simulink model "ltspidservo"  (Simulink 7.9)
settings: Solver=ode1  StartTime=0.0  StopTime=stoptime  FixedStep=(1/10000)  RelTol=1e-3
values from neighbouring files (symbols this model uses):
  Ap = [0              Cy           0          0 ... (first row only)    [LoadnCheckModel.m]
  Ayaw = [0            Cx        0           0 ... (first row only)    [LoadnCheckModel.m]
  Bp = [0 0 0 KsEL*CwEL/tausEL]'    [LoadnCheckModel.m]
  Byaw = [0     0    0   KsAZ*CwAZ/tausAZ]'    [LoadnCheckModel.m]
  Cp = [1 0 0 0]    [LoadnCheckModel.m]
  Cyaw = [1 0 0 0]    [LoadnCheckModel.m]
  dt = 0.0001    [main (ADMIN-PC's conflicted copy 2013-10-01).m]    (also in main.m)
  Gp = [0      1/Jey    0           0]'    [LoadnCheckModel.m]
  Gyaw = [0      1/Ja    0           0]'    [LoadnCheckModel.m]
  ref = 15.15    [main (ADMIN-PC's conflicted copy 2013-10-01).m]    (also in main.m)
  W = 1e-3    (= 0.001)    [main (ADMIN-PC's conflicted copy 2013-10-01).m]    (also in main.m; run_kCC.m = 1)
libraries: simulink x2
settings Model: Creator=Firdous  LastModifiedBy=ADMIN
settings DataIOCC: LimitDataPoints=off
settings GRTTargetCC: CombineOutputUpdateFcns=off  GRTInterface=on

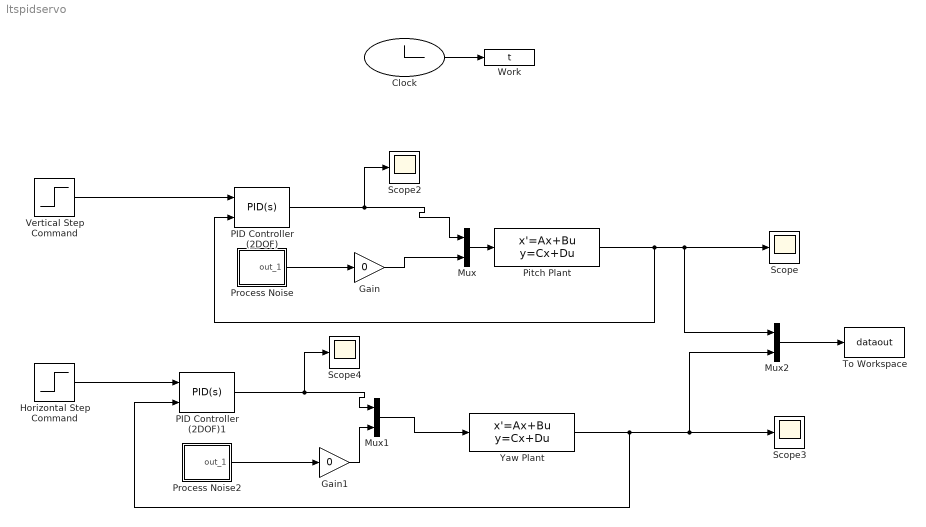
== system ltspidservo ==
  Clock : Clock
  Gain : Gain  Gain=0
  Gain1 : Gain  Gain=0
  Horizontal Step Command : Step  Time=0  After=15.15  SampleTime=0
  Mux : Mux  Inputs=2
  Mux1 : Mux  Inputs=2
  Mux2 : Mux  Inputs=2
  PID Controller (2DOF) : simulink/Continuous/PID Controller (2DOF)  Controller=PID  TimeDomain=Continuous-time  SampleTime=1  IntegratorMethod=Forward Euler  FilterMethod=Forward Euler  Form=Parallel  P=0.0314639161164997  I=0.00100652390344052  D=0.118069343591076  N=9.02659370005772  b=1  c=1  InitialConditionSource=internal  InitialConditionForIntegrator=0  InitialConditionForFilter=0  ExternalReset=none  LimitOutput=off  UpperSaturationLimit=inf  LowerSaturationLimit=-inf  LinearizeAsGain=off  AntiWindupMode=none  Kb=1  TrackingMode=off  Kt=1  PParamMin=[]  PParamMax=[]  IParamMin=[]  IParamMax=[]  DParamMin=[]  DParamMax=[]  NParamMin=[]  NParamMax=[]  bParamMin=[]  bParamMax=[]  cParamMin=[]  cParamMax=[]  KbParamMin=[]  KbParamMax=[]  KtParamMin=[]  KtParamMax=[]  POutMin=[]  POutMax=[]  IOutMin=[]  IOutMax=[]  DOutMin=[]  DOutMax=[]  NOutMin=[]  NOutMax=[]  bOutMin=[]  bOutMax=[]  cOutMin=[]  cOutMax=[]  KbOutMin=[]  KbOutMax=[]  KtOutMin=[]  KtOutMax=[]  IntegratorOutMin=[]  IntegratorOutMax=[]  FilterOutMin=[]  FilterOutMax=[]  SumOutMin=[]  SumOutMax=[]  Sum1OutMin=[]  Sum1OutMax=[]  Sum2OutMin=[]  Sum2OutMax=[]  Sum3OutMin=[]  Sum3OutMax=[]  SumI1OutMin=[]  SumI1OutMax=[]  SumI2OutMin=[]  SumI2OutMax=[]  SumI3OutMin=[]  SumI3OutMax=[]  SumDOutMin=[]  SumDOutMax=[]  SaturationOutMin=[]  SaturationOutMax=[]  IntegratorContinuousStateAttributes=''  IntegratorStateMustResolveToSignalObject=off  IntegratorRTWStateStorageClass=Auto  FilterContinuousStateAttributes=''  FilterStateMustResolveToSignalObject=off  FilterRTWStateStorageClass=Auto
  PID Controller (2DOF)1 : simulink/Continuous/PID Controller (2DOF)  Controller=PID  TimeDomain=Continuous-time  SampleTime=1  IntegratorMethod=Forward Euler  FilterMethod=Forward Euler  Form=Parallel  P=0.0104040475760461  I=0.000243006668049098  D=0.0472971950488125  N=6.44927650740255  b=1  c=1  InitialConditionSource=internal  InitialConditionForIntegrator=0  InitialConditionForFilter=0  ExternalReset=none  LimitOutput=off  UpperSaturationLimit=inf  LowerSaturationLimit=-inf  LinearizeAsGain=off  AntiWindupMode=none  Kb=1  TrackingMode=off  Kt=1  PParamMin=[]  PParamMax=[]  IParamMin=[]  IParamMax=[]  DParamMin=[]  DParamMax=[]  NParamMin=[]  NParamMax=[]  bParamMin=[]  bParamMax=[]  cParamMin=[]  cParamMax=[]  KbParamMin=[]  KbParamMax=[]  KtParamMin=[]  KtParamMax=[]  POutMin=[]  POutMax=[]  IOutMin=[]  IOutMax=[]  DOutMin=[]  DOutMax=[]  NOutMin=[]  NOutMax=[]  bOutMin=[]  bOutMax=[]  cOutMin=[]  cOutMax=[]  KbOutMin=[]  KbOutMax=[]  KtOutMin=[]  KtOutMax=[]  IntegratorOutMin=[]  IntegratorOutMax=[]  FilterOutMin=[]  FilterOutMax=[]  SumOutMin=[]  SumOutMax=[]  Sum1OutMin=[]  Sum1OutMax=[]  Sum2OutMin=[]  Sum2OutMax=[]  Sum3OutMin=[]  Sum3OutMax=[]  SumI1OutMin=[]  SumI1OutMax=[]  SumI2OutMin=[]  SumI2OutMax=[]  SumI3OutMin=[]  SumI3OutMax=[]  SumDOutMin=[]  SumDOutMax=[]  SaturationOutMin=[]  SaturationOutMax=[]  IntegratorContinuousStateAttributes=''  IntegratorStateMustResolveToSignalObject=off  IntegratorRTWStateStorageClass=Auto  FilterContinuousStateAttributes=''  FilterStateMustResolveToSignalObject=off  FilterRTWStateStorageClass=Auto
  Pitch Plant : StateSpace  A=Ap  B=[Bp Gp]  C=Cp  D=zeros(1,2)  X0=[2 0 0 0]
  Process Noise : Subsystem  mask(Continuous White Noise.){Cov=W, Ts=dt, seed=[23341]}
      mask prompts: Cov "Noise Variance:"; Ts "Sample Time:"
      mask help:
      | White noise for continuous (s-domain) systems.
      | Band-limited using zero-order-hold.
      mask Help: Implemented using white noise into Zero Order Hold block. For faster simulation set sample time to highest value possible but in accordance with the fastest dynamics of system.
      mask Display: plot(1:20,rand(size(1:20)))
  Process Noise2 : Subsystem  mask(Continuous White Noise.){Cov=W, Ts=dt, seed=[23341]}
      mask prompts: Cov "Noise Variance:"; Ts "Sample Time:"
      mask help:
      | White noise for continuous (s-domain) systems.
      | Band-limited using zero-order-hold.
      mask Help: Implemented using white noise into Zero Order Hold block. For faster simulation set sample time to highest value possible but in accordance with the fastest dynamics of system.
      mask Display: plot(1:20,rand(size(1:20)))
  Scope{,2..4} (4 alike) : Scope
      Scope settings: YMin=14.9  YMax=15.5
      Scope2 settings: YMin=17  YMax=31  SaveName=ScopeData2
      Scope3 settings: YMin=14.2  YMax=15.9  SaveName=ScopeData3
      Scope4 settings: YMin=17  YMax=31  SaveName=ScopeData4
  To Workspace : ToWorkspace  VariableName=dataout  SampleTime=-1
  Vertical Step Command : Step  Time=0  After=ref  SampleTime=0
  Work : ToWorkspace  VariableName=t
  Yaw Plant : StateSpace  A=Ayaw  B=[Byaw Gyaw]  C=Cyaw  D=zeros(1,2)  X0=[2 0 0 0]
  wires:
  Clock/1 -> Work/1
  Pitch Plant/1 -> PID Controller (2DOF)/2, Scope/1, Mux2/1
  Vertical Step Command/1 -> PID Controller (2DOF)/1
  Mux/1 -> Pitch Plant/1
  PID Controller (2DOF)/1 -> Scope2/1, Mux/1
  Process Noise/1(out_1) -> Gain/1
  Gain/1 -> Mux/2
  Yaw Plant/1 -> PID Controller (2DOF)1/2, Scope3/1, Mux2/2
  Horizontal Step Command/1 -> PID Controller (2DOF)1/1
  Mux1/1 -> Yaw Plant/1
  PID Controller (2DOF)1/1 -> Scope4/1, Mux1/1
  Process Noise2/1(out_1) -> Gain1/1
  Gain1/1 -> Mux1/2
  Mux2/1 -> To Workspace/1

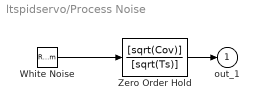
== system ltspidservo/Process Noise ==
  White Noise : RandomNumber  Seed=seed  SampleTime=dt
  Zero Order Hold : DiscreteTransferFcn  Numerator=[sqrt(Cov)]  Denominator=[sqrt(Ts)]  SampleTime=Ts
  out_1 : Outport
  wires:
  Zero Order Hold/1 -> out_1/1
  White Noise/1 -> Zero Order Hold/1

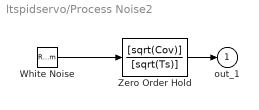
== system ltspidservo/Process Noise2 ==
  White Noise : RandomNumber  Seed=seed  SampleTime=dt
  Zero Order Hold : DiscreteTransferFcn  Numerator=[sqrt(Cov)]  Denominator=[sqrt(Ts)]  SampleTime=Ts
  out_1 : Outport
  wires:
  Zero Order Hold/1 -> out_1/1
  White Noise/1 -> Zero Order Hold/1
